simulink model "eqestate"  (R2024a)
settings: Solver=ode45  StartTime=0.0  StopTime=100  FixedStep=0.001  RelTol=1e-3  EnableMultiTasking=on
undefined symbols (not defined in the file): Adaptive_controler, ControlFeedback, deg, Equation_state_quat, Error_quaternio, InitialCondition, Ley_adaptacion, rad, s
libraries: aerolibconvert2 x12, sharedtransform x6, aerolibanim x3, aerolibtransform2 x1
settings Model: Creator=Brayan  LastModifiedBy=b_ant
settings SolverCC: AlgebraicLoopSolver=TrustRegion
settings DataIOCC: LimitDataPoints=on  SaveFormat=Array  ReturnWorkspaceOutputs=off
settings OptimizationCC: LifeSpan=inf
settings DebuggingCC: UnconnectedInputMsg=warning  UnconnectedOutputMsg=warning  UnconnectedLineMsg=warning  SFUnexpectedBacktrackingDiag=warning  SFNoUnconditionalDefaultTransitionDiag=warning  SFExecutionAtInitializationDiag=none  ArithmeticOperatorsInVariantConditions=warning
settings HardwareCC: ProdBitPerPointer=32  ProdBitPerSizeT=32  ProdBitPerPtrDiffT=32  ProdLargestAtomicFloat=None  ProdIntDivRoundTo=Undefined  ProdEndianess=Unspecified  ProdWordSize=32  ProdHWDeviceType=32-bit Generic
settings ModelReferenceCC: PropagateSignalLabelsOutOfModel=off
settings SFSimCC: SimUseLocalCustomCode=off  CustomCodeUndefinedFunction=UseInterfaceOnly
settings RTWCC: RTWUseLocalCustomCode=off  GPUComputeCapability=3.5
settings CodeAppCC: StateflowObjectComments=on
settings GRTTargetCC: TargetLangStandard=C89/C90 (ANSI)
settings ConfigComp: CovMetricSettings=dw  CovSaveCumulativeToWorkspaceVar=on  CovSaveSingleToWorkspaceVar=on  CovExternalEMLEnable=off

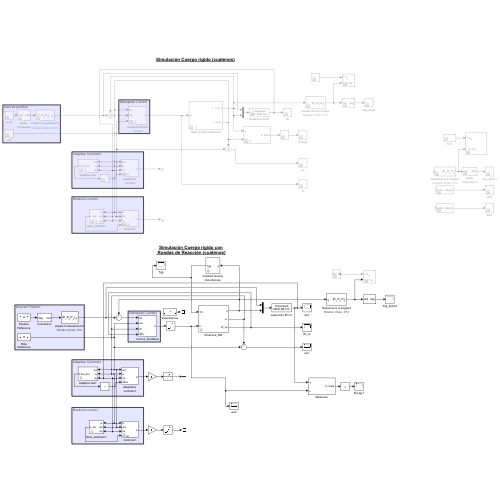
[thumbnail: Simulink's stored preview of the top-level diagram]
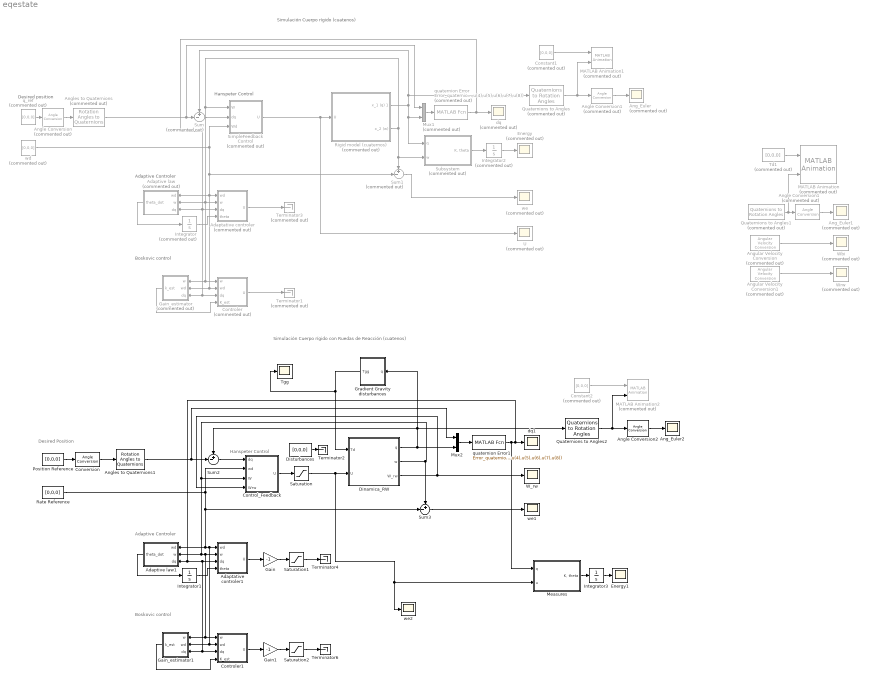
== system eqestate ==
  note: Hanspeter Control
  note: Desired Position
  note: Hanspeter Control
  note: Boskovic control
  note: Desired position
  note: Adaptive Controler
  note: Simulación Cuerpo rígido (cuatenos)
  note: Simulación Cuerpo rígido con
      | Ruedas de Reacción (cuatenos)
  note: Adaptive Controler
  note: Boskovic control
  Adaptative controler : Subsystem  Commented=on  mask{J=[1,1,1,0,0,0], lambda=10, kd=100}
      mask prompts: J "[Jcxx,Jcyy,Jczz,Jcxy,Jcxz,Jcyz]:"
      mask TypeOptions J: J/Value
      mask TypeOptions lambda: lambda/Value
      mask TypeOptions kd: Kd/Value
      mask DialogControl DescGroupVar Prompt: Adaptive controler
      mask DialogControl Control2 Prompt: Modeled inertia tensor:
      mask DialogControl H Prompt: Gains
  Adaptative controler1 : Subsystem  mask{J=[1,1,1,0,0,0], lambda=1, kd=1}
      mask prompts: J "[Jcxx,Jcyy,Jczz,Jcxy,Jcxz,Jcyz]:"
      mask TypeOptions J: J/Value
      mask TypeOptions lambda: lambda/Value
      mask TypeOptions kd: Kd/Value
      mask DialogControl DescGroupVar Prompt: Adaptive controler
      mask DialogControl Control2 Prompt: Modeled inertia tensor:
      mask DialogControl H Prompt: Gains
  Adaptive law : Subsystem  Commented=on  mask{gamma=0.01, Lambda=10}
      mask TypeOptions gamma: gamma/Value
      mask TypeOptions Lambda: lambda/Value
  Adaptive law1 : Subsystem  mask{gamma=0.001, Lambda=1}
      mask TypeOptions gamma: gamma/Value
      mask TypeOptions Lambda: lambda/Value
  Ang_Euler : Scope  Commented=on
  Ang_Euler1 : Scope  Commented=on
  Ang_Euler2 : Scope
  Angle Conversion : aerolibconvert2/Angle Conversion  Commented=on  IU=deg  OU=rad
  Angle Conversion1 : aerolibconvert2/Angle Conversion  Commented=on  IU=rad  OU=deg
  Angle Conversion1 : aerolibconvert2/Angle Conversion  Commented=on  IU=rad  OU=deg
  Angle Conversion2 : aerolibconvert2/Angle Conversion  IU=rad  OU=deg
  Angles to Quaternions : sharedtransform/Rotation Angles to Quaternions  Commented=on  rotationOrder=ZYX  aMode=aMode
  Angles to Quaternions1 : sharedtransform/Rotation Angles to Quaternions  rotationOrder=ZYX  aMode=aMode
  Angular Velocity Conversion : aerolibconvert2/Angular Velocity Conversion  Commented=on  IU=rad/s  OU=deg/s
  Angular Velocity Conversion1 : aerolibconvert2/Angular Velocity Conversion  Commented=on  IU=rad/s  OU=deg/s
  Constant1 : Constant  Commented=on  Value=[0,0,0]
  Constant2 : Constant  Commented=on  Value=[0,0,0]
  Control_Feedback : Subsystem  mask{Inertia=[1,1,1,0,0,0], P=1, K=0.5, dimentios=[0.01,0.020,0.04]}
      mask prompts: Inertia "[Ix,Iy,Iz,Ixy,Ixz,Iyz]:"; dimentios "[Grosor,Masa,Radio]:"
      mask TypeOptions Inertia: I/Value
      mask TypeOptions P: P/Value
      mask TypeOptions K: K/Value
      mask TypeOptions dimentios: dimentions/Value
      mask DialogControl ParameterGroupVar Prompt: Feedback Control
      mask DialogControl Control3 Prompt: Gains
      mask DialogControl Container2 Prompt: Reaction wheels
      mask DialogControl Control2 Prompt: Dimentions:
  Controler : Subsystem  Commented=on  mask{delta=0.005, Umax=2.3258}
      mask TypeOptions delta: delta/Value
      mask TypeOptions Umax: Umax/Value
      mask DialogControl DescGroupVar Prompt: Boskovic Control
      mask DialogControl Control2 Prompt: Delta:
      mask DialogControl Control3 Prompt: Umax:
  Controler1 : Subsystem  mask{delta=1, Umax=1.343*10^(-2)}
      mask TypeOptions delta: delta/Value
      mask TypeOptions Umax: Umax/Value
      mask DialogControl DescGroupVar Prompt: Boskovic Control
      mask DialogControl Control2 Prompt: Delta:
      mask DialogControl Control3 Prompt: Umax:
  Conversion : aerolibconvert2/Angle Conversion  IU=deg  OU=rad
  Dinamica_RW : Subsystem  mask{I=[8.46,8.46,8.46,1.1,1.5,1.6]*10^(-3), Ang=[30,0,-30], W=[0,0,30], Wrw=[0,0,30], dimensiones=[0.015,0.025,0.043]}
      mask prompts: I "[Ix,Iy,Iz,Ixy,Ixz,Iyz] :"; Ang "[roll,pitch,yaw]:"; W "[Wx,Wy,Wz]"; Wrw "[Wrwx,Wrwy,Wrwz]"; dimensiones "[Ancho,Masa,Radio]:"
      mask TypeOptions I: I/Value
      mask TypeOptions Ang: Ang/Value
      mask TypeOptions W: W/Value
      mask TypeOptions Wrw: Wrw/Value
      mask TypeOptions dimensiones: dimentions/Value
      mask DialogControl Container3 Prompt: Tensor de Inercia
      mask DialogControl Container2 Prompt: Condiciones iniciales
      mask DialogControl Container4 Prompt: Ruedas de Reacción:
      mask DialogControl Control1 Prompt: Dimensiones:
  Disturbances : Constant  Value=[0,0,0]
  Energy : Scope  Commented=on
  Energy1 : Scope
  Gain : Gain  Gain=-1
  Gain1 : Gain  Gain=-1
  Gain_estimator : Subsystem  Commented=on  mask{delta=0.005, gamma=0.01, Umax=2.3258, InitialCondition=1}
      mask prompts: InitialCondition "Simulink:blkprm_prompts:IntegratorInitCond"
      mask TypeOptions delta: delta/Value
      mask TypeOptions gamma: gamma/Value
      mask TypeOptions Umax: Umax/Value
      mask TypeOptions InitialCondition: Integrator/InitialCondition
      mask DialogControl DescGroupVar Prompt: Gain_estimator
      mask DialogControl Control2 Prompt: Gains:
      mask DialogControl Control3 Prompt: Initial Gain:
      mask DialogControl InitialCondition Prompt: Initial condition:
  Gain_estimator1 : Subsystem  mask{delta=1, gamma=0.001, Umax=1.343*10^(-2), InitialCondition=1}
      mask prompts: InitialCondition "Simulink:blkprm_prompts:IntegratorInitCond"
      mask TypeOptions delta: delta/Value
      mask TypeOptions gamma: gamma/Value
      mask TypeOptions Umax: Umax/Value
      mask TypeOptions InitialCondition: Integrator/InitialCondition
      mask DialogControl DescGroupVar Prompt: Gain_estimator
      mask DialogControl Control2 Prompt: Gains:
      mask DialogControl Control3 Prompt: Initial Gain:
      mask DialogControl InitialCondition Prompt: Initial condition:
  Gradient Gravity disturbances : Subsystem  mask{J_tilde=[8.46,8.46,8.46,1.1,1.5,1.6]*10^(-3), rc=(6371+100)*10^(3), Drw=[0.015,0.025,0.043]}
      mask prompts: J_tilde "Satellite Inertia Tensor:"; rc "Distance from the center of the earth:"; Drw "Reaction wheels dimentions"
      mask TypeOptions J_tilde: J_tilde/Value
      mask TypeOptions rc: rc/Value
      mask TypeOptions Drw: dimentions/Value
      mask DialogControl DescGroupVar Prompt: Gravity gradient Torque
  Integrator : Integrator  Commented=on  InitialCondition=[1,1,1,0,0,0]
  Integrator1 : Integrator  InitialCondition=[1,1,1,0,0,0]
  Integrator2 : Integrator  Commented=on
  Integrator3 : Integrator
  MATLAB Animation : aerolibanim/MATLAB Animation  Tag=Matlab Animation 6 DOF  Commented=on  Vehicles=1  Geometries='astredwedge.mat'  BoundingBoxCoordinates=[-50,50,-50,50,-50,50]  CameraOffset=[-150,-50,0]  CameraViewAngle=3  SampleTime=0.2  FigurePosition=[685,42,681,669]
  MATLAB Animation1 : aerolibanim/MATLAB Animation  Tag=Matlab Animation 6 DOF  Commented=on  Vehicles=1  Geometries='ac3d_xyzisrgb.ac'  BoundingBoxCoordinates=[-50,50,-50,50,-50,50]  CameraOffset=[-150,-50,0]  CameraViewAngle=3  SampleTime=0.2  FigurePosition=[685,42,681,669]
  MATLAB Animation2 : aerolibanim/MATLAB Animation  Tag=Matlab Animation 6 DOF  Commented=on  Vehicles=1  Geometries='ac3d_xyzisrgb.ac'  BoundingBoxCoordinates=[-50,50,-50,50,-50,50]  CameraOffset=[-150,-50,0]  CameraViewAngle=3  SampleTime=0.2  FigurePosition=[962,-270,958,722]
  Measures : Subsystem
  Mux1 : Mux  Commented=on  Inputs=2
  Mux2 : Mux  Inputs=2
  Position Reference : Constant  Value=[0,0,0]
  Quaternions to Angles : sharedtransform/Quaternions to Rotation Angles  Commented=on  rotationOrder=ZYX  aMode=aMode
  Quaternions to Angles1 : sharedtransform/Quaternions to Rotation Angles  Commented=on  rotationOrder=ZYX  aMode=aMode
  Quaternions to Angles2 : sharedtransform/Quaternions to Rotation Angles  rotationOrder=ZYX  aMode=aMode
  Rate Reference : Constant  Value=[0,0,0]
  Rigid model (cuaternos) : Subsystem  Commented=on  mask{I=[8.46,8.46,8.46,1.1,1.5,1.6], Value=[0,0,30], Wo=[0,0,0]}
      mask prompts: I "[Ixx,Iyy,Izz,Ixy,Ixz,Iyz] :"; Value "[roll,pitch,yaw]:"; Wo "[W0_x,W0_y,W0_z]:"
      mask TypeOptions I: I/Value
      mask TypeOptions Value: qo/Value
      mask TypeOptions Wo: Wo/Value
      mask DialogControl ParameterGroupVar Prompt: Dinamica Cuaternos
      mask DialogControl Control2 Prompt: Tensor de inercia:
      mask DialogControl Control1 Prompt: Condiciones iniciales:
  Saturation : Saturate  UpperLimit=1.343*10^(-2)  LowerLimit=-1.343*10^(-2)
  Saturation1 : Saturate  UpperLimit=1.343*10^(-2)  LowerLimit=-1.343*10^(-2)
  Saturation2 : Saturate  UpperLimit=1.343*10^(-2)  LowerLimit=-1.343*10^(-2)
  SimpleFeedback Control : Subsystem  Commented=on  mask{I=[1,1,1,0,0,0], K=1, P=10}
      mask prompts: I "[Ixx,Iyy,Izz,Ixy,Ixz,Iyz] :"
      mask TypeOptions I: I/Value
      mask TypeOptions K: K/Value
      mask TypeOptions P: P/Value
      mask DialogControl Control2 Prompt: Tensor de inercia:
      mask DialogControl Control4 Prompt: Gains
  Subsystem : Subsystem  Commented=on  mask{Value=[8.46,8.46,8.46,1.1,1.5,1.6]}
      mask prompts: Value "Inertia tensor"
      mask TypeOptions Value: J/Value
      mask DialogControl DescGroupVar Prompt: Measure of inertia and displacement
  Sum : Sum  Commented=on  Inputs=+-|
  Sum1 : Sum  Commented=on  Inputs=+-|
  Sum2 : Sum  Inputs=+-|
  Sum3 : Sum  Inputs=+-|
  Td1 : Constant  Commented=on  Value=[0,0,0]
  Terminator1 : Terminator  Commented=on
  Terminator2 : Terminator
  Terminator3 : Terminator  Commented=on
  Terminator4 : Terminator
  Terminator6 : Terminator
  Tgg : Scope
  U : Scope  Commented=on
  W_rw : Scope
  Wbi : Scope  Commented=on
  "Wrw " : Scope  Commented=on
  dq : Scope  Commented=on
  dq1 : Scope
  q_ref : Constant  Commented=on  Value=[0,0,0]
  quaternion Error : MATLABFcn  Commented=on  MATLABFcn=Error_quaternio(u(1),u(2),u(3),u(4),u(5),u(6),u(7),u(8))
  quaternion Error1 : MATLABFcn  MATLABFcn=Error_quaternio(u(1),u(2),u(3),u(4),u(5),u(6),u(7),u(8))
  wd : Constant  Commented=on  Value=[0,0,0]
  we : Scope  Commented=on
  we1 : Scope
  we2 : Scope
  wires:
  Constant1/1 -> MATLAB Animation1/1
  q_ref/1 -> Angle Conversion/1
  Angle Conversion/1 -> Angles to Quaternions/1
  Angle Conversion1/1 -> Ang_Euler/1
  Sum/1 -> SimpleFeedback Control/2(dq)
  Quaternions to Angles/1 -> Angle Conversion1/1, MATLAB Animation1/2
  Rigid model (cuaternos)/1(x_1 (q) 1) -> Subsystem/1(q), Mux1/2, Sum/1, Quaternions to Angles/1
  Mux1/1 -> quaternion Error/1
  Angles to Quaternions/1 -> Mux1/1, Sum/2
  Adaptive law/1(theta_dot) -> Integrator/1
  Integrator/1 -> Adaptative controler/4(theta)
  quaternion Error/1 -> dq/1, Controler/3(dq), Gain_estimator/3(dq), Adaptive law/3(dq), Adaptative controler/3(dq)
  wd/1 -> Controler/2(wd), Gain_estimator/2(wd), Adaptive law/1(wd), Adaptative controler/1(wd), Sum1/2, SimpleFeedback Control/3(Wd)
  Sum1/1 -> we/1
  Rigid model (cuaternos)/2("x_2 (w) ") -> SimpleFeedback Control/1(W), Adaptive law/2(w), Gain_estimator/1(w), Controler/1(w), Adaptative controler/2(w), Sum1/1, Subsystem/2(w)
  Gain_estimator/1(k_est) -> Controler/4(K_est)
  Quaternions to Angles1/1 -> Angle Conversion1/1, MATLAB Animation/2
  Angle Conversion1/1 -> Ang_Euler1/1
  Angular Velocity Conversion/1 -> Wbi/1
  Angular Velocity Conversion1/1 -> "Wrw "/1
  Td1/1 -> MATLAB Animation/1
  Dinamica_RW/3(W_rw) -> Control_Feedback/4(Wrw), W_rw/1
  Sum2/1 -> Control_Feedback/1(dq)
  Conversion/1 -> Angles to Quaternions1/1
  Position Reference/1 -> Conversion/1
  Angles to Quaternions1/1 -> Sum2/2, Mux2/1
  Adaptive law1/1(theta_dot) -> Integrator1/1
  Integrator1/1 -> Adaptative controler1/4(theta)
  Mux2/1 -> quaternion Error1/1
  Sum3/1 -> we1/1
  Constant2/1 -> MATLAB Animation2/1
  Angle Conversion2/1 -> Ang_Euler2/1
  Quaternions to Angles2/1 -> MATLAB Animation2/2, Angle Conversion2/1
  SimpleFeedback Control/1(U) -> U/1, Rigid model (cuaternos)/1(U)
  Adaptative controler/1(U) -> Terminator3/1
  quaternion Error1/1 -> Measures/1(q), Controler1/3(dq), Gain_estimator1/3(dq), Adaptative controler1/3(dq), Adaptive law1/3(dq), dq1/1
  Rate Reference/1 -> Controler1/2(wd), Gain_estimator1/2(wd), Adaptative controler1/1(wd), Adaptive law1/1(wd), Sum3/2, Control_Feedback/2(wd)
  Gain_estimator1/1(k_est) -> Controler1/4(K_est)
  Subsystem/1("K, theta") -> Integrator2/1
  Integrator2/1 -> Energy/1
  Controler/1(U) -> Terminator1/1
  Adaptative controler1/1(U) -> Gain/1
  Controler1/1(U) -> Gain1/1
  Dinamica_RW/1(q) -> Mux2/2, Gradient Gravity disturbances/1(q), Quaternions to Angles2/1, Sum2/1
  Dinamica_RW/2("w ") -> Adaptative controler1/2(w), Controler1/1(w), Gain_estimator1/1(w), Adaptive law1/2(w), Control_Feedback/3(W), Sum3/1
  Measures/1("K, theta") -> Integrator3/1
  Gain/1 -> Saturation1/1
  Gain1/1 -> Saturation2/1
  Control_Feedback/1(U) -> Saturation/1
  Integrator3/1 -> Energy1/1
  Gradient Gravity disturbances/1(Tgg) -> Tgg/1, Dinamica_RW/1(Td)
  Disturbances/1 -> Terminator2/1
  Saturation2/1 -> Terminator6/1
  Saturation1/1 -> Terminator4/1
  Saturation/1 -> Measures/2(u), we2/1, Dinamica_RW/2(U)

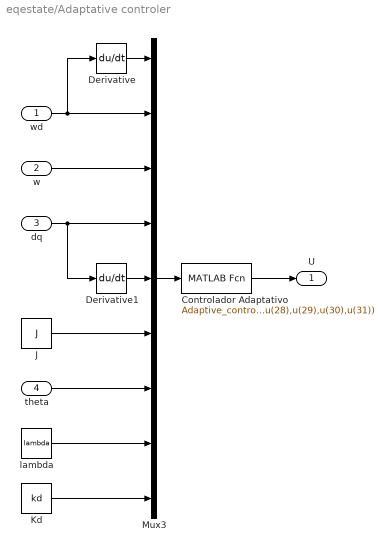
== system eqestate/Adaptative controler ==
  wd : Inport
  w : Inport  Port=2
  dq : Inport  Port=3
  theta : Inport  Port=4
  Controlador Adaptativo : MATLABFcn  MATLABFcn=Adaptive_controler(u(1),u(2),u(3),u(4),u(5),u(6),u(7),u(8),u(9),u(10),u(11),u(12),u(13),u(14),u(15),u(16),u(17),u(18),u(19),u(20),u(21),u(22),u(23),u(24),u(25),u(26),u(27),u(28),u(29),u(30),u(31))
  Derivative : Derivative
  Derivative1 : Derivative
  J : Constant  Value=J
  Kd : Constant  Value=kd
  Mux3 : Mux  Inputs=9
  lambda : Constant  Value=lambda
  U : Outport
  wires:
  Mux3/1 -> Controlador Adaptativo/1
  Controlador Adaptativo/1 -> U/1
  Derivative/1 -> Mux3/1
  Kd/1 -> Mux3/9
  wd/1 -> Derivative/1, Mux3/2
  w/1 -> Mux3/3
  dq/1 -> Derivative1/1, Mux3/4
  Derivative1/1 -> Mux3/5
  J/1 -> Mux3/6
  theta/1 -> Mux3/7
  lambda/1 -> Mux3/8

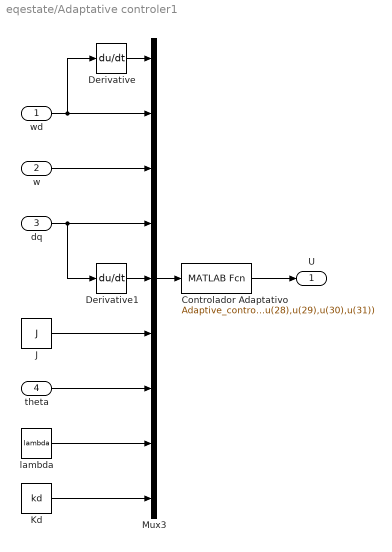
== system eqestate/Adaptative controler1 ==
  wd : Inport
  w : Inport  Port=2
  dq : Inport  Port=3
  theta : Inport  Port=4
  Controlador Adaptativo : MATLABFcn  MATLABFcn=Adaptive_controler(u(1),u(2),u(3),u(4),u(5),u(6),u(7),u(8),u(9),u(10),u(11),u(12),u(13),u(14),u(15),u(16),u(17),u(18),u(19),u(20),u(21),u(22),u(23),u(24),u(25),u(26),u(27),u(28),u(29),u(30),u(31))
  Derivative : Derivative
  Derivative1 : Derivative
  J : Constant  Value=J
  Kd : Constant  Value=kd
  Mux3 : Mux  Inputs=9
  lambda : Constant  Value=lambda
  U : Outport
  wires:
  Mux3/1 -> Controlador Adaptativo/1
  Controlador Adaptativo/1 -> U/1
  Derivative/1 -> Mux3/1
  Kd/1 -> Mux3/9
  wd/1 -> Derivative/1, Mux3/2
  w/1 -> Mux3/3
  dq/1 -> Derivative1/1, Mux3/4
  Derivative1/1 -> Mux3/5
  J/1 -> Mux3/6
  theta/1 -> Mux3/7
  lambda/1 -> Mux3/8

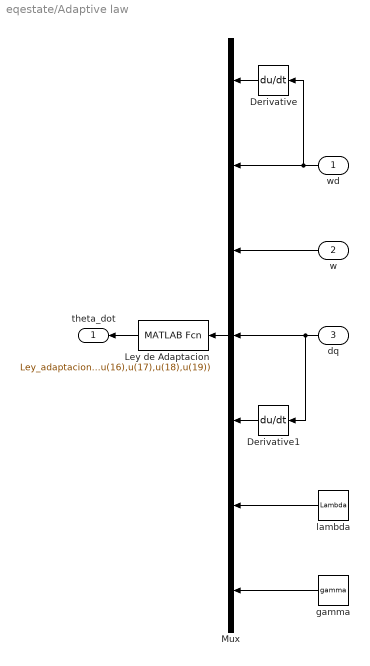
== system eqestate/Adaptive law ==
  wd : Inport
  w : Inport  Port=2
  dq : Inport  Port=3
  Derivative : Derivative
  Derivative1 : Derivative
  Ley de Adaptacion : MATLABFcn  MATLABFcn=Ley_adaptacion(u(1),u(2),u(3),u(4),u(5),u(6),u(7),u(8),u(9),u(10),u(11),u(12),u(13),u(14),u(15),u(16),u(17),u(18),u(19))
  Mux : Mux  Inputs=7
  gamma : Constant  Value=gamma
  lambda : Constant  Value=Lambda
  theta_dot : Outport
  wires:
  wd/1 -> Derivative/1, Mux/2
  Mux/1 -> Ley de Adaptacion/1
  Ley de Adaptacion/1 -> theta_dot/1
  w/1 -> Mux/3
  dq/1 -> Derivative1/1, Mux/4
  Derivative1/1 -> Mux/5
  lambda/1 -> Mux/6
  gamma/1 -> Mux/7
  Derivative/1 -> Mux/1

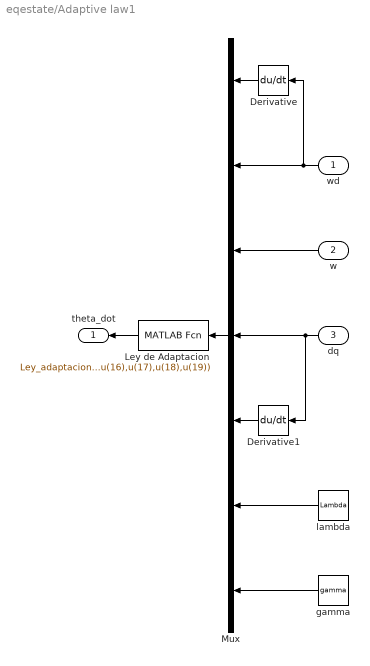
== system eqestate/Adaptive law1 ==
  wd : Inport
  w : Inport  Port=2
  dq : Inport  Port=3
  Derivative : Derivative
  Derivative1 : Derivative
  Ley de Adaptacion : MATLABFcn  MATLABFcn=Ley_adaptacion(u(1),u(2),u(3),u(4),u(5),u(6),u(7),u(8),u(9),u(10),u(11),u(12),u(13),u(14),u(15),u(16),u(17),u(18),u(19))
  Mux : Mux  Inputs=7
  gamma : Constant  Value=gamma
  lambda : Constant  Value=Lambda
  theta_dot : Outport
  wires:
  wd/1 -> Derivative/1, Mux/2
  Mux/1 -> Ley de Adaptacion/1
  Ley de Adaptacion/1 -> theta_dot/1
  w/1 -> Mux/3
  dq/1 -> Derivative1/1, Mux/4
  Derivative1/1 -> Mux/5
  lambda/1 -> Mux/6
  gamma/1 -> Mux/7
  Derivative/1 -> Mux/1

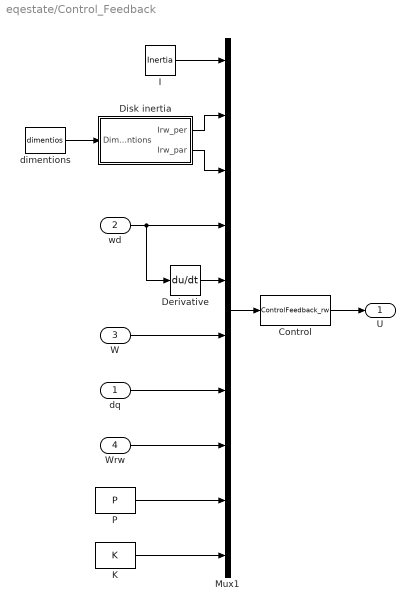
== system eqestate/Control_Feedback ==
  dq : Inport
  wd : Inport  Port=2
  W : Inport  Port=3
  Wrw : Inport  Port=4
  Control : MATLABFcn  MATLABFcn=ControlFeedback_rw
  Derivative : Derivative
  Disk inertia : Subsystem
  I : Constant  Value=Inertia
  K : Constant  Value=K
  Mux1 : Mux  Inputs=10
  P : Constant  Value=P
  dimentions : Constant  Value=dimentios
  U : Outport
  wires:
  Derivative/1 -> Mux1/5
  Mux1/1 -> Control/1
  I/1 -> Mux1/1
  Control/1 -> U/1
  W/1 -> Mux1/6
  Wrw/1 -> Mux1/8
  dq/1 -> Mux1/7
  wd/1 -> Derivative/1, Mux1/4
  dimentions/1 -> Disk inertia/1(Dimentions)
  Disk inertia/1(Irw_per) -> Mux1/2
  Disk inertia/2(Irw_par) -> Mux1/3
  K/1 -> Mux1/10
  P/1 -> Mux1/9

== system eqestate/Controler ==
  w : Inport
  wd : Inport  Port=2
  dq : Inport  Port=3
  K_est : Inport  Port=4
  Boskovic_control : MATLABFcn  MATLABFcn=Boskovic_control
  Mux : Mux  Inputs=6
  Umax : Constant  Value=Umax
  delta : Constant  Value=delta
  U : Outport
  wires:
  Boskovic_control/1 -> U/1
  Mux/1 -> Boskovic_control/1
  Umax/1 -> Mux/6
  K_est/1 -> Mux/5
  delta/1 -> Mux/4
  dq/1 -> Mux/3
  wd/1 -> Mux/2
  w/1 -> Mux/1

== system eqestate/Controler1 ==
  w : Inport
  wd : Inport  Port=2
  dq : Inport  Port=3
  K_est : Inport  Port=4
  Boskovic_control : MATLABFcn  MATLABFcn=Boskovic_control
  Mux : Mux  Inputs=6
  Umax : Constant  Value=Umax
  delta : Constant  Value=delta
  U : Outport
  wires:
  Boskovic_control/1 -> U/1
  Mux/1 -> Boskovic_control/1
  Umax/1 -> Mux/6
  K_est/1 -> Mux/5
  delta/1 -> Mux/4
  dq/1 -> Mux/3
  wd/1 -> Mux/2
  w/1 -> Mux/1

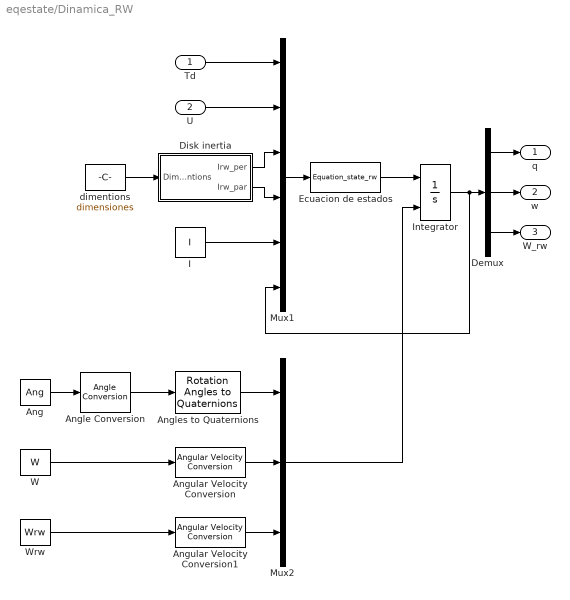
== system eqestate/Dinamica_RW ==
  Td : Inport
  U : Inport  Port=2
  Ang : Constant  Value=Ang
  Angle Conversion : aerolibconvert2/Angle Conversion  IU=deg  OU=rad
  Angles to Quaternions : sharedtransform/Rotation Angles to Quaternions  rotationOrder=ZYX  aMode=aMode
  Angular Velocity Conversion : aerolibconvert2/Angular Velocity Conversion  IU=deg/s  OU=rad/s
  Angular Velocity Conversion1 : aerolibconvert2/Angular Velocity Conversion  IU=deg/s  OU=rad/s
  Demux : Demux  Outputs=3
  Disk inertia : Subsystem
  Ecuacion de estados : MATLABFcn  MATLABFcn=Equation_state_rw
  I : Constant  Value=I
  Integrator : Integrator  InitialConditionSource=external  InitialCondition=InitialCondition
  Mux1 : Mux  Inputs=6
  Mux2 : Mux  Inputs=3
  W : Constant  Value=W
  Wrw : Constant  Value=Wrw
  dimentions : Constant  Value=dimensiones
  q : Outport
  "w " : Outport  Port=2
  W_rw : Outport  Port=3
  wires:
  Demux/1 -> q/1
  Demux/3 -> W_rw/1
  Demux/2 -> "w "/1
  Td/1 -> Mux1/1
  Ecuacion de estados/1 -> Integrator/1
  Mux1/1 -> Ecuacion de estados/1
  U/1 -> Mux1/2
  I/1 -> Mux1/5
  Mux2/1 -> Integrator/2
  Angular Velocity Conversion1/1 -> Mux2/3
  Angular Velocity Conversion/1 -> Mux2/2
  Angle Conversion/1 -> Angles to Quaternions/1
  Ang/1 -> Angle Conversion/1
  Wrw/1 -> Angular Velocity Conversion1/1
  Angles to Quaternions/1 -> Mux2/1
  Integrator/1 -> Mux1/6, Demux/1
  W/1 -> Angular Velocity Conversion/1
  dimentions/1 -> Disk inertia/1(Dimentions)
  Disk inertia/1(Irw_per) -> Mux1/3
  Disk inertia/2(Irw_par) -> Mux1/4

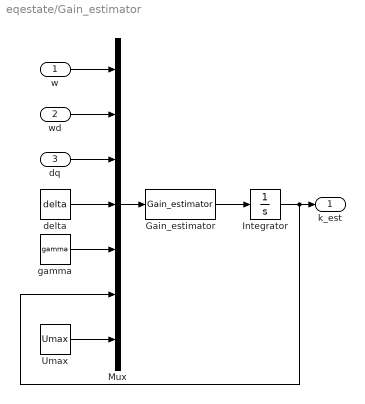
== system eqestate/Gain_estimator ==
  w : Inport
  wd : Inport  Port=2
  dq : Inport  Port=3
  Gain_estimator : MATLABFcn  MATLABFcn=Gain_estimator
  Integrator : Integrator  InitialCondition=InitialCondition
  Mux : Mux  Inputs=7
  Umax : Constant  Value=Umax
  delta : Constant  Value=delta
  gamma : Constant  Value=gamma
  k_est : Outport
  wires:
  Gain_estimator/1 -> Integrator/1
  Mux/1 -> Gain_estimator/1
  Integrator/1 -> Mux/6, k_est/1
  Umax/1 -> Mux/7
  gamma/1 -> Mux/5
  delta/1 -> Mux/4
  dq/1 -> Mux/3
  wd/1 -> Mux/2
  w/1 -> Mux/1

== system eqestate/Gain_estimator1 ==
  w : Inport
  wd : Inport  Port=2
  dq : Inport  Port=3
  Gain_estimator : MATLABFcn  MATLABFcn=Gain_estimator
  Integrator : Integrator  InitialCondition=InitialCondition
  Mux : Mux  Inputs=7
  Umax : Constant  Value=Umax
  delta : Constant  Value=delta
  gamma : Constant  Value=gamma
  k_est : Outport
  wires:
  Gain_estimator/1 -> Integrator/1
  Mux/1 -> Gain_estimator/1
  Integrator/1 -> Mux/6, k_est/1
  Umax/1 -> Mux/7
  gamma/1 -> Mux/5
  delta/1 -> Mux/4
  dq/1 -> Mux/3
  wd/1 -> Mux/2
  w/1 -> Mux/1

== system eqestate/Gradient Gravity disturbances ==
  q : Inport
  Disk inertia : Subsystem
  Gravity disturbances : MATLABFcn  MATLABFcn=T_disturbances
  J_tilde : Constant  Value=J_tilde
  Mux3 : Mux
  Terminator2 : Terminator
  dimentions : Constant  Value=Drw
  rc : Constant  Value=rc
  Tgg : Outport
  wires:
  dimentions/1 -> Disk inertia/1(Dimentions)
  rc/1 -> Mux3/3
  J_tilde/1 -> Mux3/1
  Mux3/1 -> Gravity disturbances/1
  Disk inertia/1(Irw_per) -> Mux3/4
  Disk inertia/2(Irw_par) -> Terminator2/1
  q/1 -> Mux3/2
  Gravity disturbances/1 -> Tgg/1

== system eqestate/Measures ==
  q : Inport
  u : Inport  Port=2
  Measure : MATLABFcn  MATLABFcn=Measures
  Mux3 : Mux  Inputs=2
  "K, theta" : Outport
  wires:
  Measure/1 -> "K, theta"/1
  Mux3/1 -> Measure/1
  q/1 -> Mux3/1
  u/1 -> Mux3/2

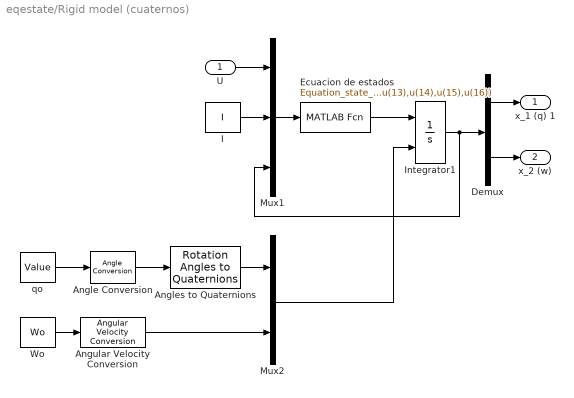
== system eqestate/Rigid model (cuaternos) ==
  U : Inport
  Angle Conversion : aerolibconvert2/Angle Conversion  IU=deg  OU=rad
  Angles to Quaternions : aerolibtransform2/Rotation Angles to Quaternions  rotationOrder=ZYX
  Angular Velocity Conversion : aerolibconvert2/Angular Velocity Conversion  IU=deg/s  OU=rad/s
  Demux : Demux  Outputs=2
  Ecuacion de estados : MATLABFcn  MATLABFcn=Equation_state_quat(u(1),u(2),u(3),u(4),u(5),u(6),u(7),u(8),u(9),u(10),u(11),u(12),u(13),u(14),u(15),u(16))
  I : Constant  Value=I
  Integrator1 : Integrator  InitialConditionSource=external  InitialCondition=[1,0,0,0,0.5,0.1,0.2]
  Mux1 : Mux  Inputs=3
  Mux2 : Mux  Inputs=2
  Wo : Constant  Value=Wo
  qo : Constant  Value=Value
  x_1 (q) 1 : Outport
  "x_2 (w) " : Outport  Port=2
  wires:
  Demux/1 -> x_1 (q) 1/1
  Integrator1/1 -> Mux1/3, Demux/1
  Demux/2 -> "x_2 (w) "/1
  U/1 -> Mux1/1
  Mux1/1 -> Ecuacion de estados/1
  I/1 -> Mux1/2
  Mux2/1 -> Integrator1/2
  Angles to Quaternions/1 -> Mux2/1
  Angle Conversion/1 -> Angles to Quaternions/1
  qo/1 -> Angle Conversion/1
  Wo/1 -> Angular Velocity Conversion/1
  Angular Velocity Conversion/1 -> Mux2/2
  Ecuacion de estados/1 -> Integrator1/1

== system eqestate/SimpleFeedback Control ==
  W : Inport
  dq : Inport  Port=2
  Wd : Inport  Port=3
  Derivative : Derivative
  I : Constant  Value=I
  K : Constant  Value=K
  Mux2 : Mux  Inputs=7
  P : Constant  Value=P
  Simple Feedback Control : MATLABFcn  MATLABFcn=ControlFeedback(u(1),u(2),u(3),u(4),u(5),u(6),u(7),u(8),u(9),u(10),u(11),u(12),u(13),u(14),u(15),u(16),u(17),u(18),u(19),u(20),u(21))
  U : Outport
  wires:
  Wd/1 -> Derivative/1, Mux2/2
  I/1 -> Mux2/1
  Mux2/1 -> Simple Feedback Control/1
  Simple Feedback Control/1 -> U/1
  dq/1 -> Mux2/5
  W/1 -> Mux2/4
  K/1 -> Mux2/7
  P/1 -> Mux2/6
  Derivative/1 -> Mux2/3

== system eqestate/Subsystem ==
  q : Inport
  w : Inport  Port=2
  J : Constant  Value=Value
  Measure : MATLABFcn  MATLABFcn=Measures
  Mux3 : Mux  Inputs=3
  "K, theta" : Outport
  wires:
  J/1 -> Mux3/3
  w/1 -> Mux3/2
  q/1 -> Mux3/1
  Mux3/1 -> Measure/1
  Measure/1 -> "K, theta"/1

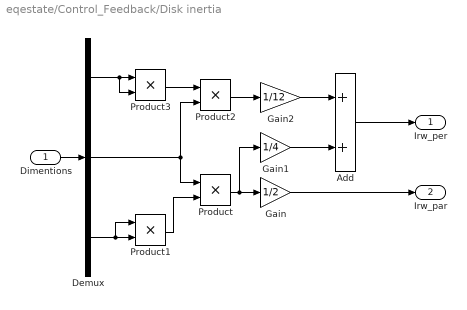
== system eqestate/Control_Feedback/Disk inertia ==
  Dimentions : Inport
  Add : Sum
  Demux : Demux  Outputs=3
  Gain : Gain  Gain=1/2
  Gain1 : Gain  Gain=1/4
  Gain2 : Gain  Gain=1/12
  Product{,1..3} (4 alike) : Product
  Irw_per : Outport
  Irw_par : Outport  Port=2
  wires:
  Product3/1 -> Product2/1
  Gain2/1 -> Add/1
  Product/1 -> Gain1/1, Gain/1
  Add/1 -> Irw_per/1
  Gain1/1 -> Add/2
  Product1/1 -> Product/2
  Gain/1 -> Irw_par/1
  Demux/1 -> Product3/2, Product3/1
  Product2/1 -> Gain2/1
  Demux/2 -> Product/1, Product2/2
  Dimentions/1 -> Demux/1
  Demux/3 -> Product1/1, Product1/2

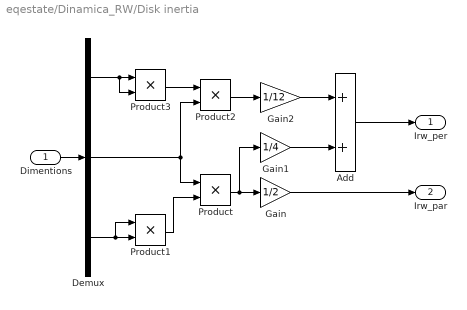
== system eqestate/Dinamica_RW/Disk inertia ==
  Dimentions : Inport
  Add : Sum
  Demux : Demux  Outputs=3
  Gain : Gain  Gain=1/2
  Gain1 : Gain  Gain=1/4
  Gain2 : Gain  Gain=1/12
  Product{,1..3} (4 alike) : Product
  Irw_per : Outport
  Irw_par : Outport  Port=2
  wires:
  Product3/1 -> Product2/1
  Gain2/1 -> Add/1
  Product/1 -> Gain1/1, Gain/1
  Add/1 -> Irw_per/1
  Gain1/1 -> Add/2
  Product1/1 -> Product/2
  Gain/1 -> Irw_par/1
  Demux/1 -> Product3/2, Product3/1
  Product2/1 -> Gain2/1
  Demux/2 -> Product/1, Product2/2
  Dimentions/1 -> Demux/1
  Demux/3 -> Product1/1, Product1/2

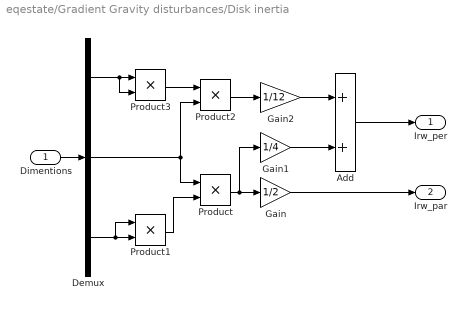
== system eqestate/Gradient Gravity disturbances/Disk inertia ==
  Dimentions : Inport
  Add : Sum
  Demux : Demux  Outputs=3
  Gain : Gain  Gain=1/2
  Gain1 : Gain  Gain=1/4
  Gain2 : Gain  Gain=1/12
  Product{,1..3} (4 alike) : Product
  Irw_per : Outport
  Irw_par : Outport  Port=2
  wires:
  Product3/1 -> Product2/1
  Gain2/1 -> Add/1
  Product/1 -> Gain1/1, Gain/1
  Add/1 -> Irw_per/1
  Gain1/1 -> Add/2
  Product1/1 -> Product/2
  Gain/1 -> Irw_par/1
  Demux/1 -> Product3/2, Product3/1
  Product2/1 -> Gain2/1
  Demux/2 -> Product/1, Product2/2
  Dimentions/1 -> Demux/1
  Demux/3 -> Product1/1, Product1/2
